simulink library "wakeEffect_ul"  (R2022a)
settings: Solver=VariableStepAuto  StartTime=0.0  StopTime=10.0  RelTol=1e-3
undefined symbols (not defined in the file): aeroStruct, vhcl
settings Model: Creator=adabney  LastModifiedBy=adabney

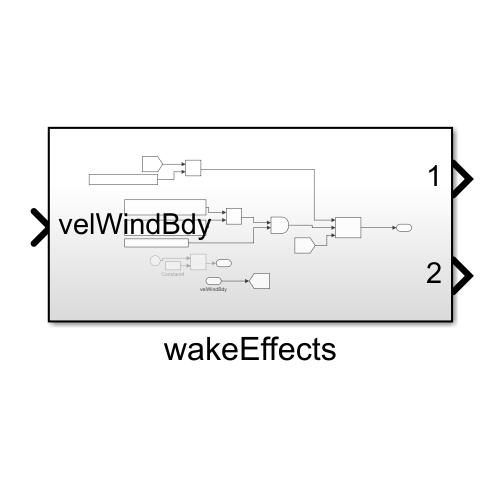
[thumbnail: Simulink's stored preview of the top-level diagram]
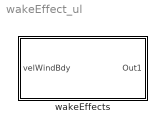
== system wakeEffect_ul ==
  wakeEffects : Subsystem

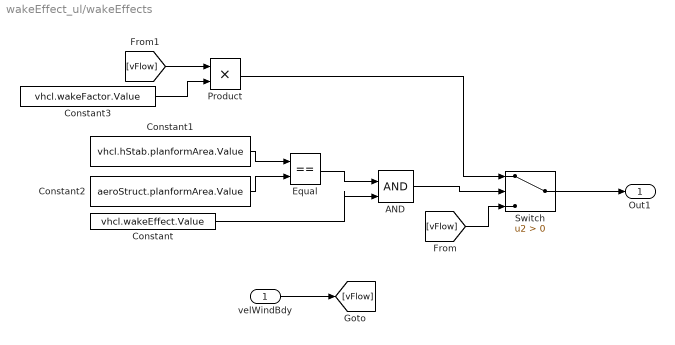
== system wakeEffect_ul/wakeEffects ==
  velWindBdy : Inport
  AND : Logic  IconShape=distinctive  AllPortsSameDT=off  OutDataTypeStr=boolean
  Constant : Constant  Value=vhcl.wakeEffect.Value
  Constant1 : Constant  Value=vhcl.hStab.planformArea.Value
  Constant2 : Constant  Value=aeroStruct.planformArea.Value
  Constant3 : Constant  Value=vhcl.wakeFactor.Value
  Equal : RelationalOperator  Operator===  OutDataTypeStr=boolean  RndMeth=Simplest  InputSameDT=off
  Product : Product
  Switch : Switch  Criteria=u2 > Threshold  SaturateOnIntegerOverflow=off  InputSameDT=off
  Out1 : Outport
  wires:
  Constant/1 -> AND/2
  Constant2/1 -> Equal/2
  velWindBdy/1 -> [vFlow]
  Product/1 -> Switch/1
  Switch/1 -> Out1/1
  AND/1 -> Switch/2
  [vFlow] -> Product/1
  Constant1/1 -> Equal/1
  Equal/1 -> AND/1
  [vFlow] -> Switch/3
  Constant3/1 -> Product/2
